simulink subsystem "refuel_GS_N2_subsystem"  (R2025a)
settings: Solver=VariableStepAuto  StartTime=0.0  StopTime=10.0  RelTol=1e-3
undefined symbols (not defined in the file): AC_engine_feed_pipe_length, AC_engine_feed_port_inner_diameter, GroundAmbientTemp_K, GS_Hose_Length_m, GS_Hose_MassPerLength_kgpm, GS_Hose_SurfaceAreaPerLength, GS_Initial_Pressurant_Temp_K, wall_thickness
libraries: fl_lib x8, nesl_utility x3, SimscapeFluids_lib x1
settings Model: Creator=MW  LastModifiedBy=MW

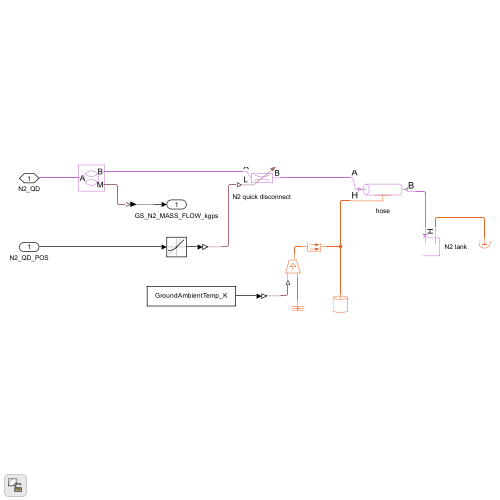
[thumbnail: Simulink's stored preview of the top-level diagram]
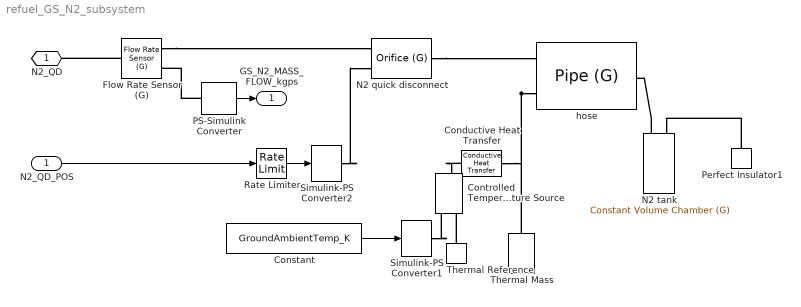
== system refuel_GS_N2_subsystem ==
  N2_QD_POS : Inport
  Conductive Heat Transfer : fl_lib/Thermal/Thermal Elements/Conductive Heat Transfer  thermal_type=foundation.enum.ConstantVariableTabulated.Constant  wall_geometry=foundation.enum.ConductionWallGeometry.Planar  area=GS_Hose_SurfaceAreaPerLength*GS_Hose_Length_m m^2  thickness=GS_Hose_Thickness_m m  d_in=AC_engine_feed_port_inner_diameter m  d_out=wall_thickness*2 + AC_engine_feed_port_inner_diameter m  L=AC_engine_feed_pipe_length m  th_cond_min=10 W/(K*m)  th_cond=Ally_conductivity_Wpmk W/(m*K)  th_cond_TLU=[413, 401, 392, 383, 371, 357, 342] W/(K*m)  temp_TLU=[200, 273, 400, 600, 800, 1000, 1200] K  T_specify=off  T_priority=None  T=0 K  T_nominal_specify=off  T_nominal_value=1  T_nominal_unit=K  Q_specify=off  Q_priority=None  Q=0 W  Q_nominal_specify=off  Q_nominal_value=1  Q_nominal_unit=W
  Constant : Constant  Value=GroundAmbientTemp_K
  Controlled Temperature Source : fl_lib/Thermal/Thermal Sources/Controlled Temperature Source
  Flow Rate Sensor (G) : fl_lib/Gas/Sensors/Flow Rate Sensor (G)  mass_flow_measure=true  volumetric_flow_measure=false  volumetric_flow_conditions=foundation.enum.volumetric_flow_conditions.actual  p_std=0.101325 MPa  T_std=20 degC  energy_flow_measure=false
      settings: InternalSimscapePortConfiguration="{\"Bottom\":[],\"Left\":[{\"id\":\"A\",\"label\":\"A\",\"type\":\"foundation.gas.gas\"}],\"Right\":[{\"id\":\"B\",\"label\":\"B\",\"type\":\"foundation.gas.gas\"},{\"id\":\"M\",\"label\":\"M\",\"type\":\"output\"}],\"Top\":[]}"
  N2 quick disconnect : SimscapeFluids_lib/Gas/Valves & Orifices/Orifice (G)  orifice_type=foundation.enum.constant_variable.variable  orifice_parameterization=fluids.gas.valves_orifices.enum.OrificeParameterization.Area  opening_characteristic=fluids.gas.valves_orifices.enum.OpeningCharacteristics.Linear  Cv_constant=4  Cv_max=4  L_Cv_TLU=0 : 0.2 : 1  Cv_TLU=[1e-06, .8, 1.6, 2.4, 3.2, 4]  xT_Cv=0.7  Kv_constant=3.6  Kv_max=3.6  L_Kv_TLU=0 : 0.2 : 1  Kv_TLU=[1e-06, .72, 1.44, 2.16, 2.88, 3.6]  xT_Kv=0.7  C_constant=12 l/(bar*s)  B_crit_constant=0.3  C_max=12 l/(bar*s)  B_crit_linear=0.3  L_C_TLU=0 : 0.2 : 1  C_TLU=[1e-05, 2.4, 4.8, 7.2, 9.6, 12] l/(bar*s)  B_crit_TLU=0.3 * ones(1, 6)  m=0.5  T_ref_C=293.15 K  rho_ref_C=1.185 kg/m^3  orifice_area_constant=1e-4 m^2  orifice_area_max=QD_OrificeArea_m2 m^2  L_orifice_area_TLU=0 : 0.2 : 1  orifice_area_TLU=[1e-10, 2e-05, 4e-05, 6e-05, 8e-05, .0001] m^2  Cd=0.64  leakage_fraction=QD_LeakageRatio  smoothing_factor=0.01  B_lam=0.999  area=Pressurant_pipe_area_m2 m^2
      settings: InternalSimscapePortConfiguration="{\"Bottom\":[],\"Left\":[{\"id\":\"A\",\"label\":\"A\",\"type\":\"foundation.gas.gas\"},{\"id\":\"L\",\"label\":\"L\",\"type\":\"input\"}],\"Right\":[{\"id\":\"B\",\"label\":\"B\",\"type\":\"foundation.gas.gas\"}],\"Top\":[]}"
  N2 tank : fl_lib/Gas/Elements/Constant Volume Chamber (G)  volume=GS_Pressurant_Tank_Volume_L l  num_ports=foundation.enum.num_ports.one  area_A=Pressurant_pipe_area_m2 m^2  area_B=0.01 m^2  area_C=0.01 m^2  area_D=0.01 m^2  p_I_specify=on  p_I_priority=High  p_I=GS_Initial_Pressurant_Pressure_bar bar  p_I_nominal_specify=on  p_I_nominal_value=GS_Initial_Pressurant_Pressure_bar  p_I_nominal_unit=bar  T_I_specify=on  T_I_priority=High  T_I=GS_Initial_Pressurant_Temp_K K  T_I_nominal_specify=off  T_I_nominal_value=1  T_I_nominal_unit=K  rho_I_specify=off  rho_I_priority=None  rho_I=1.2 kg/m^3  rho_I_nominal_specify=off  rho_I_nominal_value=1  rho_I_nominal_unit=kg/m^3
      settings: InternalSimscapePortConfiguration="{\"Bottom\":[],\"Left\":[{\"id\":\"A\",\"label\":\"A\",\"type\":\"foundation.gas.gas\"},{\"id\":\"H\",\"label\":\"H\",\"type\":\"foundation.thermal.thermal\"}],\"Right\":[],\"Top\":[]}"
  PS-Simulink Converter : nesl_utility/PS-Simulink Converter  PhysicalDomain=network_engine_domain  SubClassName=ps_output  LeftPortType=input  RightPortType=output  PseudoPeriodic=off  Frequencies=[]  VectorFormat=inherit  Unit=inherit  AffineConversion=off
  Perfect Insulator1 : fl_lib/Thermal/Thermal Elements/Perfect Insulator  T_specify=off  T_priority=None  T=293.15 K  T_nominal_specify=off  T_nominal_value=1  T_nominal_unit=K
  Rate Limiter : RateLimiter  SampleTimeMode=inherited
  Simulink-PS Converter1 : nesl_utility/Simulink-PS Converter  PhysicalDomain=network_engine_domain  SubClassName=ps_input  LeftPortType=input  RightPortType=output  PseudoPeriodic=off  Frequencies=[]  NoiseDistribution=none  NoiseParameters=[]  Unit=1  AffineConversion=off  FilteringAndDerivatives=zero  SimscapeFilterOrder=1  InputFilterTimeConstant=0.001  UdotUserProvided=1
  Simulink-PS Converter2 : nesl_utility/Simulink-PS Converter  PhysicalDomain=network_engine_domain  SubClassName=ps_input  LeftPortType=input  RightPortType=output  PseudoPeriodic=off  Frequencies=[]  NoiseDistribution=none  NoiseParameters=[]  Unit=1  AffineConversion=off  FilteringAndDerivatives=provide  SimscapeFilterOrder=1  InputFilterTimeConstant=0.001  UdotUserProvided=0
  Thermal Mass : fl_lib/Thermal/Thermal Elements/Thermal Mass  mass_type=foundation.enum.constant_variable.constant  mass=GS_Hose_MassPerLength_kgpm*GS_Hose_Length_m kg  sp_heat=Ally_heatCapacity_Jpkgk J/kg/K  mass_min=1e-6 kg  num_ports=foundation.enum.numPorts2.one  m_specify=off  m_priority=High  m=1 kg  m_nominal_specify=off  m_nominal_value=1  m_nominal_unit=kg  T_specify=on  T_priority=High  T=GS_Initial_Pressurant_Temp_K K  T_nominal_specify=off  T_nominal_value=1  T_nominal_unit=K  Q_specify=off  Q_priority=None  Q=0 W  Q_nominal_specify=off  Q_nominal_value=1  Q_nominal_unit=W
  Thermal Reference : fl_lib/Thermal/Thermal Elements/Thermal Reference
  hose : fl_lib/Gas/Elements/Pipe (G)  length=GS_Hose_Length_m m  area=Pressurant_pipe_area_m2 m^2  Dh=Pressurant_pipe_diameter_m m  length_add=0.1 m  roughness=15e-6 m  Re_lam=2000  Re_tur=4000  shape_factor=64  Nu_lam=3.66  dynamic_compressibility=true  inertia=false  p_init=GS_Initial_Pressurant_Pressure_bar bar  p_init_priority=foundation.enum.Priority.High  T_init=GS_Initial_Pressurant_Temp_K K  T_init_priority=foundation.enum.Priority.High  mdot_init=0 kg/s  mdot_init_priority=foundation.enum.Priority.High  p_nominal=0.101325 MPa  T_nominal=293.15 K
  N2_QD : PMIOPort  Side=Left
  GS_N2_MASS_FLOW_kgps : Outport
  wires:
  N2_QD_POS/1 -> Rate Limiter/1
  PS-Simulink Converter/1 -> GS_N2_MASS_FLOW_kgps/1
  Rate Limiter/1 -> Simulink-PS Converter2/1
  Constant/1 -> Simulink-PS Converter1/1
  connections:
  hose/LConn2 -- Conductive Heat Transfer/RConn1 -- Thermal Mass/LConn1
  N2 quick disconnect/RConn1 -- hose/LConn1
  Simulink-PS Converter2/RConn1 -- N2 quick disconnect/LConn2
  Flow Rate Sensor (G)/LConn1 -- N2_QD/RConn1
  N2 tank/LConn1 -- hose/RConn1
  Flow Rate Sensor (G)/RConn1 -- N2 quick disconnect/LConn1
  PS-Simulink Converter/LConn1 -- Flow Rate Sensor (G)/RConn2
  Perfect Insulator1/LConn1 -- N2 tank/LConn2
  Thermal Reference/LConn1 -- Controlled Temperature Source/RConn2
  Conductive Heat Transfer/LConn1 -- Controlled Temperature Source/LConn1
  Simulink-PS Converter1/RConn1 -- Controlled Temperature Source/RConn1
